simulink model "simulation_lqr"  (R2014b)
settings: Solver=ode45  StartTime=0.0  StopTime=400  RelTol=1e-3
undefined symbols (not defined in the file or in its folder): K
settings Model: Creator=jonas  LastModifiedBy=jonas
settings DataIOCC: LimitDataPoints=off

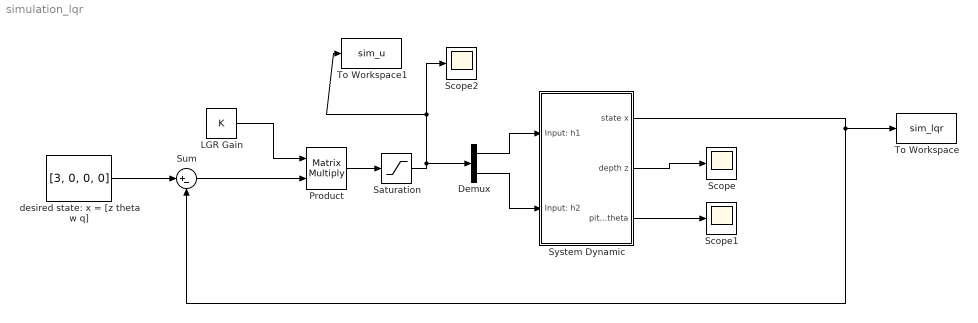
== system simulation_lqr ==
  Demux : Demux  Outputs=2
  LGR Gain : Constant  Value=K
  Product : Product  Multiplication=Matrix(*)
  Saturation : Saturate  UpperLimit=1  LowerLimit=0
  Scope : Scope
      settings: TimeRange=160  YMin=1.002147239263805  YMax=4.602147239263805
  Scope1 : Scope
  Scope2 : Scope
      settings: SaveName=ScopeData2
  Sum : Sum  Inputs=|+-
  System Dynamic : Subsystem
  To Workspace : ToWorkspace  VariableName=sim_lqr  SampleTime=0.01
  To Workspace1 : ToWorkspace  VariableName=sim_u  SampleTime=0.01
  desired state: x = [z theta w q] : Constant  Value=[3, 0, 0, 0]
  wires:
  Demux/1 -> System Dynamic/1(Input: h1)
  Demux/2 -> System Dynamic/2(Input: h2)
  desired state: x = [z theta w q]/1 -> Sum/1
  System Dynamic/2(depth z) -> Scope/1
  System Dynamic/3(pitch theta) -> Scope1/1
  LGR Gain/1 -> Product/1
  Sum/1 -> Product/2
  System Dynamic/1(state x) -> To Workspace/1, Sum/2
  Product/1 -> Saturation/1
  Saturation/1 -> Demux/1, To Workspace1/1, Scope2/1

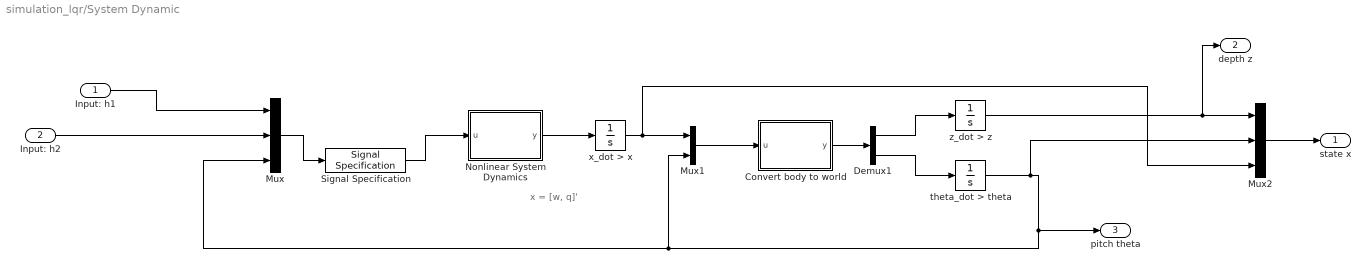
== system simulation_lqr/System Dynamic ==
  note: x = [w, q]'
  Input: h1 : Inport
  Input: h2 : Inport  Port=2
  Convert body to world : MATLAB Function  TreatAsAtomicUnit=on
  Demux1 : Demux  Outputs=2
  Mux : Mux  Inputs=3
  Mux1 : Mux  Inputs=2
  Mux2 : Mux  Inputs=3
  Nonlinear System Dynamics : MATLAB Function  TreatAsAtomicUnit=on
  Signal Specification : SignalSpecification  Dimensions=3
  theta_dot > theta : Integrator  InitialCondition=0.5
  x_dot > x : Integrator
  z_dot > z : Integrator
  state x : Outport
  depth z : Outport  Port=2
  pitch theta : Outport  Port=3
  wires:
  Convert body to world/1(y) -> Demux1/1
  Demux1/1 -> z_dot > z/1
  Demux1/2 -> theta_dot > theta/1
  z_dot > z/1 -> depth z/1, Mux2/1
  Signal Specification/1 -> Nonlinear System Dynamics/1(u)
  Mux1/1 -> Convert body to world/1(u)
  x_dot > x/1 -> Mux2/3, Mux1/1
  Mux2/1 -> state x/1
  Nonlinear System Dynamics/1(y) -> x_dot > x/1
  Mux/1 -> Signal Specification/1
  Input: h1/1 -> Mux/1
  Input: h2/1 -> Mux/2
  theta_dot > theta/1 -> Mux2/2, pitch theta/1, Mux1/2, Mux/3

== matlab function simulation_lqr/System Dynamic/Convert body to world ==
  data: u input; y output
function y = fcn(u)

x_body = [u(1), u(2)]'; % [w, q]
theta = u(3);
% transform from body to earth frame
J = [cos(theta), 0;...
    0, 1];

y = J*x_body; % [z_dot, theta_dot]

== matlab function simulation_lqr/System Dynamic/Nonlinear System Dynamics ==
  data: u input; y output
function y = fcn(u)
%#codegen

% ---- PARAMETERS ----

g   = 9.81;                 % [m/s^2]   gravity
rho = 1000;                 % [kg/m^3]  density water

% parameters nanins specific
m0  = 5.7;                    % [kg]      empty weight Nanin
l_n = 0.514;                  % [m]       length Nanin
r_n = 0.06;                  % [m]       radius Nanin
V_n = r_n^2*pi*l_n;         % [m^3]     volume Nanin

x0_t = 0.25;                % [m]       displacement piston tank in x direction
z0_t = 0.05;                % [m]       displacement piston tank in z direction
A_t = pi*(65/(2*1000))^2;   % [m^2]     area piston tank
V_t = 250e-6;               % [m^3]     volume of piston tank
h_max = V_t/A_t;            % [m]       max height of water in piston tank

Iy0 = 0.134;                % [kgm^2]   moment of inertia around y-axis

% restoring static forces
W_r = m0*g;          % [N]       gravitational force empty
B_r = rho*g*V_n;    % [N]       buoancy restoring force

% Added mass coefficents
Z_w = -rho*V_n;             % [kg]
M_q = -1/12*rho*V_n*l_n;    % [km*m]

% ------

% rename parameters for clarification
h1 = u(1);
h2 = u(2);
theta = u(3);

% Denormalize input
h1 = h1*h_max;
h2 = h2*h_max;

u_sys = [h1, h2]';

% calculate dynamic parameters
m = m0 + rho*A_t*(h1+h2); % dynamic mass
x1 = x0_t - h1/2;         % CoG of piston tank
x2 = -(x0_t - h2/2);

z_g = 0.005;
x_g = 0;
I_y = 0;

% calculate system model matrices
M = [ m-Z_w,  -m*x_g;...
     -m*x_g, I_y-M_q];
 
g_static = [-(W_r-B_r)*cos(theta);...
            z_g*W_r*sin(theta) + x_g*W_r*cos(theta)];
        
G_dyn = g*rho*A_t*[-cos(theta), -cos(theta);...
                    sin(theta)*z0_t+cos(theta)*x1, sin(theta)*z0_t+cos(theta)*x2];
                
% calcuate state w_dot, q_dot
x_dot = M\(-g_static -G_dyn*u_sys);

% return values
y = x_dot;
